simulink model "Q7"  (R2021b)
settings: Solver=VariableStepAuto  StartTime=0.0  StopTime=50  RelTol=1e-3
values from neighbouring files (symbols this model uses):
  A = [0 0 0 1 0 0 ... (first row only)    [Lab1_code.m]
  B = [0 0 0 ... (first row only)    [Lab1_code.m]
  C = [1 0 0 0 0 0 ... (first row only)    [Lab1_code.m]
  D = [0 0 0 ... (first row only)    [Lab1_code.m]
settings Model: Creator=DSDLn  LastModifiedBy=DSDLn

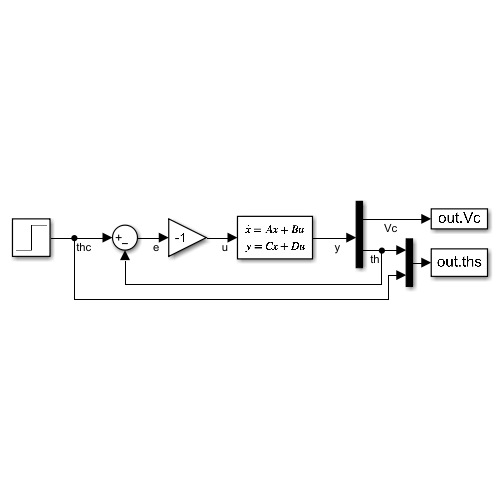
[thumbnail: Simulink's stored preview of the top-level diagram]
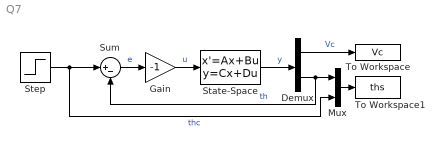
== system Q7 ==
  Demux : Demux  Outputs=2
  Gain : Gain  Gain=-1
  Mux : Mux  Inputs=2
  State-Space : StateSpace  A=A  B=B  C=C  D=D  InitialCondition=0
  Step : Step  Time=0  After=0.1  SampleTime=0
  Sum : Sum  Inputs=|+-
  To Workspace : ToWorkspace  VariableName=Vc  SampleTime=-1
  To Workspace1 : ToWorkspace  VariableName=ths  SampleTime=-1
  wires:
  Step/1 -> Mux/2, Sum/1  "thc"
  Sum/1 -> Gain/1  "e"
  Gain/1 -> State-Space/1  "u"
  State-Space/1 -> Demux/1  "y"
  Demux/1 -> To Workspace/1  "Vc"
  Demux/2 -> Mux/1, Sum/2  "th"
  Mux/1 -> To Workspace1/1
